simulink library "mbd_s32k1xx_ec_toolbox"  (Simulink 9.0)
settings: Solver=FixedStepDiscrete  StartTime=0.0  StopTime=10.0  FixedStep=0.1  RelTol=1e-3  EnableMultiTasking=on
InitFcn:
  | mbd_s32k_consistency_checks(bdroot(gcs));
(part 8 of 8)

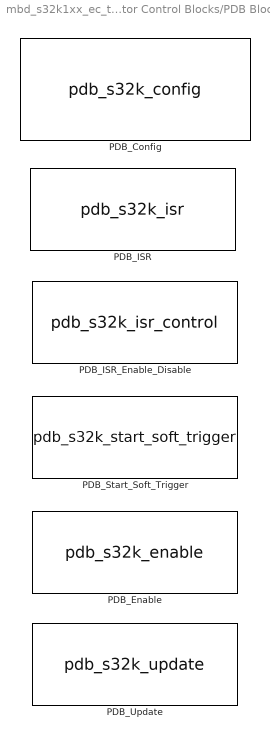
== system mbd_s32k1xx_ec_toolbox/Motor Control Blocks/PDB Blocks ==
  PDB_Config : S-Function  FunctionName=pdb_s32k_config  Parameters=funcParams  SFunctionDeploymentMode=off  EnableBusSupport=off  mask(pdb_s32k_config_block){pdbModule=0, regScCont=One-Shot, regScTrgsel=External (TRGMUX_PDB_TRIG), trgMuxSel=Trigger function is disabled, trgMuxSelPin=PTB5: [TRGMUX_IN0 | Trigger Mux Input], regModModulus=0, regScPrescaler=1, regScMult=1, regPoenPoen0=off, regPo0DlyDly1=0, regPo0DlyDly2=0, enable_pdb_init=on, show_adv_opts=on, regCh0C1En0=off, regCh0C1En1=off, regCh0C1En2=off, regCh0C1En3=off, regCh0C1En4=off, regCh0C1En5=off, regCh0C1En6=off, regCh0C1En7=off, regCh0C1Bb0=off, regCh0C1Bb1=off, regCh0C1Bb2=off, regCh0C1Bb3=off, regCh0C1Bb4=off, regCh0C1Bb5=off, regCh0C1Bb6=off, regCh0C1Bb7=off, regCh0C1Tos0=Pre-trigger is in delay mode, regCh0C1Tos1=Pre-trigger is in delay mode, regCh0C1Tos2=Pre-trigger is in delay mode, regCh0C1Tos3=Pre-trigger is in delay mode, regCh0C1Tos4=Pre-trigger is in delay mode, regCh0C1Tos5=Pre-trigger is in delay mode, regCh0C1Tos6=Pre-trigger is in delay mode, regCh0C1Tos7=Pre-trigger is in delay mode, regCh0DlyDly0=0, regCh0DlyDly1=200, regCh0DlyDly2=0, regCh0DlyDly3=0, regCh0DlyDly4=0, regCh0DlyDly5=0, regCh0DlyDly6=0, regCh0DlyDly7=0, regCh1C1En0=off, regCh1C1En1=off, regCh1C1En2=off, regCh1C1En3=off, regCh1C1En4=off, regCh1C1En5=off, regCh1C1En6=off, regCh1C1En7=off, regCh1C1Bb0=off, regCh1C1Bb1=off, regCh1C1Bb2=off, regCh1C1Bb3=off, regCh1C1Bb4=off, regCh1C1Bb5=off, regCh1C1Bb6=off, regCh1C1Bb7=off, regCh1C1Tos0=Pre-trigger is in delay mode, regCh1C1Tos1=Pre-trigger is in delay mode, regCh1C1Tos2=Pre-trigger is in delay mode, regCh1C1Tos3=Pre-trigger is in delay mode, regCh1C1Tos4=Pre-trigger is in delay mode, regCh1C1Tos5=Pre-trigger is in delay mode, regCh1C1Tos6=Pre-trigger is in delay mode, regCh1C1Tos7=Pre-trigger is in delay mode, regCh1DlyDly0=0, regCh1DlyDly1=0, regCh1DlyDly2=0, regCh1DlyDly3=0, regCh1DlyDly4=0, regCh1DlyDly5=0, regCh1DlyDly6=0, regCh1DlyDly7=0}
      mask prompts: pdbModule "Module"; regScCont "Operation Mode"; regScTrgsel "Trigger Input Source"; trgMuxSel "Input signal for External trigger"; trgMuxSelPin "Input pin for Trigger Mux Input"; regModModulus "Modulus, cycles (0 - 65535)"; regScPrescaler "Value"; regScMult "Multiplication Factor"; regPoenPoen0 "Pulse-Out0 Enable"; regPo0DlyDly1 "Pulse-Out0 Delay 1 (0 - 65535)"; regPo0DlyDly2 "Pulse-Out0 Delay 2 (0 - 65535)"; enable_pdb_init "Enable PDB in Init function"; show_adv_opts "Show Advanced Options"; regCh0C1En0 "Pre-trigger 0 Enabled"; regCh0C1En1 "Pre-trigger 1 Enabled"; regCh0C1En2 "Pre-trigger 2 Enabled"; regCh0C1En3 "Pre-trigger 3 Enabled"; regCh0C1En4 "Pre-trigger 4 Enabled"; regCh0C1En5 "Pre-trigger 5 Enabled"; regCh0C1En6 "Pre-trigger 6 Enabled"; regCh0C1En7 "Pre-trigger 7 Enabled"; regCh0C1Bb0 "Pre-trigger 0 Back-to-Back Enabled"; regCh0C1Bb1 "Pre-trigger 1 Back-to-Back Enabled"; regCh0C1Bb2 "Pre-trigger 2 Back-to-Back Enabled"; regCh0C1Bb3 "Pre-trigger 3 Back-to-Back Enabled"; regCh0C1Bb4 "Pre-trigger 4 Back-to-Back Enabled"; regCh0C1Bb5 "Pre-trigger 5 Back-to-Back Enabled"; regCh0C1Bb6 "Pre-trigger 6 Back-to-Back Enabled"; regCh0C1Bb7 "Pre-trigger 7 Back-to-Back Enabled"; regCh0C1Tos0 "Pre-Trigger 0 Output Select"; regCh0C1Tos1 "Pre-Trigger 1 Output Select"; regCh0C1Tos2 "Pre-Trigger 2 Output Select"; regCh0C1Tos3 "Pre-Trigger 3 Output Select"; regCh0C1Tos4 "Pre-Trigger 4 Output Select"; regCh0C1Tos5 "Pre-Trigger 5 Output Select"; regCh0C1Tos6 "Pre-Trigger 6 Output Select"; regCh0C1Tos7 "Pre-Trigger 7 Output Select"; regCh0DlyDly0 "Delay 0, cycles (0 - 65535)"; regCh0DlyDly1 "Delay 1, cycles (0 - 65535)"; regCh0DlyDly2 "Delay 2, cycles (0 - 65535)"; regCh0DlyDly3 "Delay 3, cycles (0 - 65535)"; regCh0DlyDly4 "Delay 4, cycles (0 - 65535)"; regCh0DlyDly5 "Delay 5, cycles (0 - 65535)"; regCh0DlyDly6 "Delay 6, cycles (0 - 65535)"; regCh0DlyDly7 "Delay 7, cycles (0 - 65535)"; regCh1C1En0 "Pre-trigger 0 Enabled"; regCh1C1En1 "Pre-trigger 1 Enabled"; regCh1C1En2 "Pre-trigger 2 Enabled"; regCh1C1En3 "Pre-trigger 3 Enabled"; regCh1C1En4 "Pre-trigger 4 Enabled"; regCh1C1En5 "Pre-trigger 5 Enabled"; regCh1C1En6 "Pre-trigger 6 Enabled"; regCh1C1En7 "Pre-trigger 7 Enabled"; regCh1C1Bb0 "Pre-trigger 0 Back-to-Back Enabled"; regCh1C1Bb1 "Pre-trigger 1 Back-to-Back Enabled"; regCh1C1Bb2 "Pre-trigger 2 Back-to-Back Enabled"; regCh1C1Bb3 "Pre-trigger 3 Back-to-Back Enabled"; regCh1C1Bb4 "Pre-trigger 4 Back-to-Back Enabled"; regCh1C1Bb5 "Pre-trigger 5 Back-to-Back Enabled"; regCh1C1Bb6 "Pre-trigger 6 Back-to-Back Enabled"; regCh1C1Bb7 "Pre-trigger 7 Back-to-Back Enabled"; regCh1C1Tos0 "Pre-Trigger 0 Output Select"; regCh1C1Tos1 "Pre-Trigger 1 Output Select"; regCh1C1Tos2 "Pre-Trigger 2 Output Select"; regCh1C1Tos3 "Pre-Trigger 3 Output Select"; regCh1C1Tos4 "Pre-Trigger 4 Output Select"; regCh1C1Tos5 "Pre-Trigger 5 Output Select"; regCh1C1Tos6 "Pre-Trigger 6 Output Select"; regCh1C1Tos7 "Pre-Trigger 7 Output Select"; regCh1DlyDly0 "Delay 0, cycles (0 - 65535)"; regCh1DlyDly1 "Delay 1, cycles (0 - 65535)"; regCh1DlyDly2 "Delay 2, cycles (0 - 65535)"; regCh1DlyDly3 "Delay 3, cycles (0 - 65535)"; regCh1DlyDly4 "Delay 4, cycles (0 - 65535)"; regCh1DlyDly5 "Delay 5, cycles (0 - 65535)"; regCh1DlyDly6 "Delay 6, cycles (0 - 65535)"; regCh1DlyDly7 "Delay 7, cycles (0 - 65535)"
      mask help: This block allows user to configure the Programmable Delay Block (PDB).
      mask init:
      | mbd_s32k_pdb_display_instances();
      | 
      | [labels, maskStr] = mbd_s32k_pdb_config_init(gcb);
      | set_param(gcb, 'MaskDisplay', labels);
      | funcParams = [];
      settings: NameChangeFcn=mbd_s32k_name_check (gcb);
      mask Help: web(fullfile(mbd_s32k_block_help, 'pdb', 'pdb_config_block.html'));
      mask TypeOptions pdbModule: 0 | 1
      mask Callback pdbModule: mbd_s32k_pdb_display_instances();
      mask TypeOptions regScCont: One-Shot | Continuous
      mask TypeOptions regScTrgsel: External (TRGMUX_PDB_TRIG) | Software
      mask Callback regScTrgsel: mbd_s32k_pdb_extrg(gcb);
      mask TypeOptions trgMuxSel: Trigger function is disabled | Trigger MUX input 0 | Trigger MUX input 1 | Trigger MUX input 2 | Trigger MUX input 3 | Trigger MUX input 4 | Trigger MUX input 5 | Trigger MUX input 6 | Trigger MUX input 7 | Trigger MUX input 8 | Trigger MUX input 9 | Trigger MUX input 10 | Trigger MUX input 11 | CMP0 Output | LPIT Channel 0 | LPIT Channel 1 | LPIT Channel 2 | LPIT Channel 3 | LPTMR0 Trigger | FTM0 Initialize Trigger | FTM0 External Trigger | FTM1 Initialize Trigger | FTM1 External Trigger | FTM2 Initialize Trigger | FTM2 External Trigger | FTM3 Initialize Trigger | FTM3 External Trigger | ADC0_COCOA | ADC0_COCOB | ADC1_COCOA | ADC1_COCOB | PDB0 Channel 0 Trigger | PDB0 Pulse out | PDB1 Channel 0 Trigger | PDB1 Pulse out | RTC Alarm | RTC Seconds Counter | Flex IO Trigger 0 | Flex IO Trigger 1 | Flex IO Trigger 2 | Flex IO Trigger 3 | LPUART0 RX Data | LPUART0 TX Data | LPUART0 RX Idle | LPUART1 RX Data | LPUART1 TX Data | LPUART1 RX Idle | LPI2C0 Master Stop | LPI2C0 Slave Stop | LPI2C1 Master Stop | LPI2C1 Slave Stop | LPSPI0 Frame | LPSPI0 RX Data | LPSPI1 Frame | LPSPI1 RX Data | SIM Software Trigger
      mask Callback trgMuxSel: mbd_s32k_pdb_extrg(gcb);
      mask TypeOptions trgMuxSelPin: PTB5: [TRGMUX_IN0 | Trigger Mux Input]
      mask Callback regModModulus: mbd_s32k_pdb_check_interval(gcb, 'regModModulus');
      mask TypeOptions regScPrescaler: 1 | 2 | 4 | 8 | 16 | 32 | 64 | 128
      mask TypeOptions regScMult: 1 | 10 | 20 | 40
      mask Callback regPoenPoen0: mbd_s32k_pdb_pulse_out_enable(gcb, '0');
      mask Callback regPo0DlyDly1: mbd_s32k_pdb_check_interval(gcb, 'regPo0DlyDly1');
      mask Callback regPo0DlyDly2: mbd_s32k_pdb_check_interval(gcb, 'regPo0DlyDly2');
      mask Callback show_adv_opts: mbd_s32k_pdb_config_cbk()
      mask Callback regCh0C1En0: mbd_s32k_pdb_channel_enable(gcb, '0', '0');
      mask Callback regCh0C1En1: mbd_s32k_pdb_channel_enable(gcb, '0', '1');
      mask Callback regCh0C1En2: mbd_s32k_pdb_channel_enable(gcb, '0', '2');
      mask Callback regCh0C1En3: mbd_s32k_pdb_channel_enable(gcb, '0', '3');
      mask Callback regCh0C1En4: mbd_s32k_pdb_channel_enable(gcb, '0', '4');
      mask Callback regCh0C1En5: mbd_s32k_pdb_channel_enable(gcb, '0', '5');
      mask Callback regCh0C1En6: mbd_s32k_pdb_channel_enable(gcb, '0', '6');
      mask Callback regCh0C1En7: mbd_s32k_pdb_channel_enable(gcb, '0', '7');
      mask TypeOptions regCh0C1Tos0: Pre-trigger is in bypassed mode | Pre-trigger is in delay mode
      mask TypeOptions regCh0C1Tos1: Pre-trigger is in bypassed mode | Pre-trigger is in delay mode
      mask TypeOptions regCh0C1Tos2: Pre-trigger is in bypassed mode | Pre-trigger is in delay mode
      mask TypeOptions regCh0C1Tos3: Pre-trigger is in bypassed mode | Pre-trigger is in delay mode
      mask TypeOptions regCh0C1Tos4: Pre-trigger is in bypassed mode | Pre-trigger is in delay mode
      mask TypeOptions regCh0C1Tos5: Pre-trigger is in bypassed mode | Pre-trigger is in delay mode
      mask TypeOptions regCh0C1Tos6: Pre-trigger is in bypassed mode | Pre-trigger is in delay mode
      mask TypeOptions regCh0C1Tos7: Pre-trigger is in bypassed mode | Pre-trigger is in delay mode
      mask Callback regCh0DlyDly0: mbd_s32k_pdb_check_interval(gcb, 'regCh0DlyDly0');
      mask Callback regCh0DlyDly1: mbd_s32k_pdb_check_interval(gcb, 'regCh0DlyDly1');
      mask Callback regCh0DlyDly2: mbd_s32k_pdb_check_interval(gcb, 'regCh0DlyDly2');
      mask Callback regCh0DlyDly3: mbd_s32k_pdb_check_interval(gcb, 'regCh0DlyDly3');
      mask Callback regCh0DlyDly4: mbd_s32k_pdb_check_interval(gcb, 'regCh0DlyDly4');
      mask Callback regCh0DlyDly5: mbd_s32k_pdb_check_interval(gcb, 'regCh0DlyDly5');
      mask Callback regCh0DlyDly6: mbd_s32k_pdb_check_interval(gcb, 'regCh0DlyDly6');
      mask Callback regCh0DlyDly7: mbd_s32k_pdb_check_interval(gcb, 'regCh0DlyDly7');
      mask Callback regCh1C1En0: mbd_s32k_pdb_channel_enable(gcb, '1', '0');
      mask Callback regCh1C1En1: mbd_s32k_pdb_channel_enable(gcb, '1', '1');
      mask Callback regCh1C1En2: mbd_s32k_pdb_channel_enable(gcb, '1', '2');
      mask Callback regCh1C1En3: mbd_s32k_pdb_channel_enable(gcb, '1', '3');
      mask Callback regCh1C1En4: mbd_s32k_pdb_channel_enable(gcb, '1', '4');
      mask Callback regCh1C1En5: mbd_s32k_pdb_channel_enable(gcb, '1', '5');
      mask Callback regCh1C1En6: mbd_s32k_pdb_channel_enable(gcb, '1', '6');
      mask Callback regCh1C1En7: mbd_s32k_pdb_channel_enable(gcb, '1', '7');
      mask TypeOptions regCh1C1Tos0: Pre-trigger is in bypassed mode | Pre-trigger is in delay mode
      mask TypeOptions regCh1C1Tos1: Pre-trigger is in bypassed mode | Pre-trigger is in delay mode
      mask TypeOptions regCh1C1Tos2: Pre-trigger is in bypassed mode | Pre-trigger is in delay mode
      mask TypeOptions regCh1C1Tos3: Pre-trigger is in bypassed mode | Pre-trigger is in delay mode
      mask TypeOptions regCh1C1Tos4: Pre-trigger is in bypassed mode | Pre-trigger is in delay mode
      mask TypeOptions regCh1C1Tos5: Pre-trigger is in bypassed mode | Pre-trigger is in delay mode
      mask TypeOptions regCh1C1Tos6: Pre-trigger is in bypassed mode | Pre-trigger is in delay mode
      mask TypeOptions regCh1C1Tos7: Pre-trigger is in bypassed mode | Pre-trigger is in delay mode
      mask Callback regCh1DlyDly0: mbd_s32k_pdb_check_interval(gcb, 'regCh1DlyDly0');
      mask Callback regCh1DlyDly1: mbd_s32k_pdb_check_interval(gcb, 'regCh1DlyDly1');
      mask Callback regCh1DlyDly2: mbd_s32k_pdb_check_interval(gcb, 'regCh1DlyDly2');
      mask Callback regCh1DlyDly3: mbd_s32k_pdb_check_interval(gcb, 'regCh1DlyDly3');
      mask Callback regCh1DlyDly4: mbd_s32k_pdb_check_interval(gcb, 'regCh1DlyDly4');
      mask Callback regCh1DlyDly5: mbd_s32k_pdb_check_interval(gcb, 'regCh1DlyDly5');
      mask Callback regCh1DlyDly6: mbd_s32k_pdb_check_interval(gcb, 'regCh1DlyDly6');
      mask Callback regCh1DlyDly7: mbd_s32k_pdb_check_interval(gcb, 'regCh1DlyDly7');
      mask DialogControl Container8 Prompt: General Settings
      mask DialogControl ParameterGroupVar0 Prompt: Prescaler Configuration
      mask DialogControl ParameterGroupVar01 Prompt: Pulse-Out Configuration
      mask Display:
      | image('nxp_logo.png', 'top-right');
      | disp(maskStr);
  PDB_Enable : S-Function  Priority=2  FunctionName=pdb_s32k_enable  SFunctionDeploymentMode=off  EnableBusSupport=off  mask(pdb_s32k_enable_block){pdbModule=0, pdbAction=Enable}
      mask prompts: pdbModule "Module"; pdbAction "Action"
      mask help: This block allows user to enable PDB block (sets PDBEN bit; if this block is not used, PDB counter is off).
      mask init:
      | maskStr = mbd_s32k_pdb_enable_to_string();
      | mbd_s32k_pdb_display_instances();
      settings: NameChangeFcn=mbd_s32k_name_check (gcb);
      mask Help: web(fullfile(mbd_s32k_block_help, 'pdb', 'pdb_enable_block.html'));
      mask TypeOptions pdbModule: 0 | 1
      mask Callback pdbModule: mbd_s32k_pdb_display_instances();
      mask TypeOptions pdbAction: Enable | Disable
      mask Display:
      | image('nxp_logo.png', 'top-right');
      | 
      | disp(maskStr);
  PDB_ISR : S-Function  Priority=2  FunctionName=pdb_s32k_isr  Parameters=funcParams  SFunctionDeploymentMode=off  EnableBusSupport=off  mask(pdb_s32k_isr_block){pdbModule=0, prioInterrupt=15, regScPdbie=off, regScPdbeie=off, regIdlyIdly=0}
      mask prompts: pdbModule "Module"; prioInterrupt "ISR priority"; regScPdbie "Counter Interrupt Enable (PDBIE)"; regScPdbeie "Sequence Error Interrupt Enable (PDBEIE)"; regIdlyIdly "Interrupt Delay, cycles (0 - 65535)"
      mask help: This block allows call user function on PDB Interrupt (when the counter value is equal to the IDLY register) or on PDB Sequence Error Interrupt.
      mask init:
      | mbd_s32k_pdb_display_instances();
      | mbd_s32k_isr_priority_cbk(gcb, 'prioInterrupt');
      | 
      | [labels, maskStr] = mbd_s32k_pdb_isr_init(gcb);
      | set_param(gcb, 'MaskDisplay', labels);
      | funcParams = [];
      settings: NameChangeFcn=mbd_s32k_name_check (gcb);
      mask Help: web(fullfile(mbd_s32k_block_help, 'pdb', 'pdb_isr_block.html'));
      mask TypeOptions pdbModule: 0 | 1
      mask Callback pdbModule: mbd_s32k_pdb_display_instances();
      mask TypeOptions prioInterrupt: 0 | 1 | 2 | 3 | 4 | 5 | 6 | 7 | 8 | 9 | 10 | 11 | 12 | 13 | 14 | 15
      mask Callback regIdlyIdly: mbd_s32k_pdb_check_interval(gcb, 'regIdlyIdly');
      mask Display:
      | image('nxp_logo.png', 'top-right');
      | port_label('output', 1, 'ISR');
      | port_label('output', 2, 'SC[PDBIF]');
      | port_label('output', 3, 'CH0S[ERRm]');
      | port_label('output', 4, 'CH1S[ERRm]');
      | disp(maskStr);
  PDB_ISR_Enable_Disable : S-Function  Priority=4  FunctionName=pdb_s32k_isr_control  Parameters=funcParams  SFunctionDeploymentMode=off  EnableBusSupport=off  mask(pdb_s32k_isr_control_block){pdbModule=0, regScPdbie=off, regScPdbeie=off}
      mask prompts: pdbModule "Module"; regScPdbie "Counter Interrupt Enable (PDBIE)"; regScPdbeie "Sequence Error Interrupt Enable (PDBEIE)"
      mask help: This block is allow to enable or disable PDB interrupts.
      mask init:
      | labels = ['image(''nxp_logo.png'', ''top-right'');', newline];
      | 
      | % Make params for s function
      | funcParams = [];
      | 
      | maskStr = [ 'PDB ISR Disable Enable Block', newline, newline, ...
      |     'Module:  ', num2str(pdbModule - 1), newline, ... 
      |     'Counter Interrupt: ', get_param(gcb,'regScPdbie'), newline, ... 
      |     'Sequence Error Interrupt: ', get_param(gcb,'regScPdbeie')];
      | 
      | mbd_s32k_pdb_display_instances();
      settings: NameChangeFcn=mbd_s32k_name_check (gcb);
      mask Help: web(fullfile(mbd_s32k_block_help, 'pdb', 'pdb_isr_control_block.html'));
      mask TypeOptions pdbModule: 0 | 1
      mask Callback pdbModule: mbd_s32k_pdb_display_instances();
      mask Display:
      | image('nxp_logo.png', 'top-right');
      | disp(maskStr);
  PDB_Start_Soft_Trigger : S-Function  Priority=3  FunctionName=pdb_s32k_start_soft_trigger  Parameters=funcParams  SFunctionDeploymentMode=off  EnableBusSupport=off  mask(pdb_s32k_start_soft_trigger_block){pdbModule=0}
      mask prompts: pdbModule "Module"
      mask help: When PDB is enabled and the software trigger is selected as the trigger input source, this block allows resets and restarts of the PDB counter.
      mask init:
      | mbd_s32k_pdb_display_instances();
      | % Make params for s function
      | funcParams = [int32(pdbModule - 1)];
      | 
      | maskStr = [ 'PDB Start Software Trigger Block', newline, newline, ...
      |     'Module:  ', num2str(pdbModule - 1)];
      settings: NameChangeFcn=mbd_s32k_name_check (gcb);
      mask Help: web(fullfile(mbd_s32k_block_help, 'pdb', 'pdb_start_soft_trigger_block.html'));
      mask TypeOptions pdbModule: 0 | 1
      mask Callback pdbModule: mbd_s32k_pdb_display_instances();
      mask Display:
      | image('nxp_logo.png', 'top-right');
      | disp(maskStr);
  PDB_Update : S-Function  Priority=2  FunctionName=pdb_s32k_update  Parameters=funcParams, funcParamNumberOfInputs  SFunctionDeploymentMode=off  EnableBusSupport=off  mask(pdb_s32k_update_block){pdbModule=0, regScLdmod=Immediately, inputModEn=off, inputIdlyEn=off, inputCh0DlyEn=off, inputCh1DlyEn=off, inputPo0DlyEn=off}
      mask prompts: pdbModule "Module"; regScLdmod "Load Mode Select"; inputModEn "Modulus input enable"; inputIdlyEn "Interrupt Delay input enable"; inputCh0DlyEn "Ch0 Delay inputs enable"; inputCh1DlyEn "Ch1 Delay inputs enable"; inputPo0DlyEn "Pulse-Out 0 Delay inputs enable"
      mask help: This block allows user to update the MOD, IDLY, CHnDLYm, INTx, and POyDLY registers, after 1 is written to LDOK.
      mask init:
      | mbd_s32k_pdb_display_instances();
      | 
      | [labels, maskStr, funcParamNumberOfInputs] = mbd_s32k_pdb_update_init(gcb);
      | set_param(gcb, 'MaskDisplay', labels);
      | funcParams = [];
      settings: NameChangeFcn=mbd_s32k_name_check (gcb);
      mask Help: web(fullfile(mbd_s32k_block_help, 'pdb', 'pdb_update_block.html'));
      mask TypeOptions pdbModule: 0 | 1
      mask Callback pdbModule: mbd_s32k_pdb_display_instances();
      mask TypeOptions regScLdmod: Immediately | PDB counter reaches the MOD register value | Trigger input event is detected | PDB counter reaches the MOD register value or a trigger input event is detected
      mask Display:
      | image('nxp_logo.png', 'top-right');
      | disp(maskStr);

== system mbd_s32k1xx_ec_toolbox/Communication Blocks/FlexIO Blocks /FlexIO I2C Blocks ==
  "FlexIO_I2C_Master_Config " : S-Function  FunctionName=flexio_i2c_master_s32k_config  SFunctionDeploymentMode=off  EnableBusSupport=off  mask(flexio_i2c_s32k_master_config){InstanceNumber=0, DriverType=Polling, BaudRate=0, SDA_pin=PTD0: [FXIO_D0 | FlexIO Bi-directional Shift/timer I/O], SCL_pin=PTD1: [FXIO_D1 | FlexIO Bi-directional Shift/timer I/O]}
      mask prompts: InstanceNumber "Instance"; DriverType "Mode"; BaudRate "Baud Rate"; SDA_pin "SDA pin"; SCL_pin "SCL pin"
      mask help: This block allows the user to configure the FlexIO module to emulate I2C communication (master mode).
      mask init:
      | maskStr = mbd_s32k_flexio_i2c_master_string();
      | mbd_s32k_flexio_i2c_master_pin_display();
      settings: NameChangeFcn=mbd_s32k_name_check(gcb);
      mask Help: web(fullfile(mbd_s32k_block_help, 'flexio', 'flexio_i2c_master_config.html'));
      mask TypeOptions InstanceNumber: 0 | 1
      mask Callback InstanceNumber: mbd_s32k_flexio_i2c_master_pin_display();
      mask TypeOptions DriverType: Polling | Interrupts
      mask TypeOptions SDA_pin: PTA10: [FXIO_D0 | FlexIO Bi-directional Shift/timer I/O] | PTA21: [FXIO_D0 | FlexIO Bi-directional Shift/timer I/O] | PTC30: [FXIO_D0 | FlexIO Bi-directional Shift/timer I/O] | PTD0: [FXIO_D0 | FlexIO Bi-directional Shift/timer I/O] | PTD9: [FXIO_D0 | FlexIO Bi-directional Shift/timer I/O] | PTA11: [FXIO_D1 | FlexIO Bi-directional Shift/timer I/O] | PTA22: [FXIO_D1 | FlexIO Bi-directional Shift/timer I/O] | PTC31: [FXIO_D1 | FlexIO Bi-directional Shift/timer I/O] | PTD1: [FXIO_D1 | FlexIO Bi-directional Shift/timer I/O] | PTD8: [FXIO_D1 | FlexIO Bi-directional Shift/timer I/O] | PTA0: [FXIO_D2 | FlexIO Bi-directional Shift/timer I/O] | PTA23: [FXIO_D2 | FlexIO Bi-directional Shift/timer I/O] | PTD18: [FXIO_D2 | FlexIO Bi-directional Shift/timer I/O] | PTE15: [FXIO_D2 | FlexIO Bi-directional Shift/timer I/O] | PTA1: [FXIO_D3 | FlexIO Bi-directional Shift/timer I/O] | PTA24: [FXIO_D3 | FlexIO Bi-directional Shift/timer I/O] | PTD19: [FXIO_D3 | FlexIO Bi-directional Shift/timer I/O] | PTE16: [FXIO_D3 | FlexIO Bi-directional Shift/timer I/O] | PTA2: [FXIO_D4 | FlexIO Bi-directional Shift/timer I/O] | PTD2: [FXIO_D4 | FlexIO Bi-directional Shift/timer I/O] | PTE10: [FXIO_D4 | FlexIO Bi-directional Shift/timer I/O] | PTE18: [FXIO_D4 | FlexIO Bi-directional Shift/timer I/O] | PTA3: [FXIO_D5 | FlexIO Bi-directional Shift/timer I/O] | PTD3: [FXIO_D5 | FlexIO Bi-directional Shift/timer I/O] | PTE11: [FXIO_D5 | FlexIO Bi-directional Shift/timer I/O] | PTE17: [FXIO_D5 | FlexIO Bi-directional Shift/timer I/O] | PTA8: [FXIO_D6 | FlexIO Bi-directional Shift/timer I/O] | PTD2: [FXIO_D6 | FlexIO Bi-directional Shift/timer I/O] | PTD31: [FXIO_D6 | FlexIO Bi-directional Shift/timer I/O] | PTE4: [FXIO_D6 | FlexIO Bi-directional Shift/timer I/O] | PTA9: [FXIO_D7 | FlexIO Bi-directional Shift/timer I/O] | PTD3: [FXIO_D7 | FlexIO Bi-directional Shift/timer I/O] | PTD26: [FXIO_D7 | FlexIO Bi-directional Shift/timer I/O] | PTE5: [FXIO_D7 | FlexIO Bi-directional Shift/timer I/O]
      mask TypeOptions SCL_pin: PTA10: [FXIO_D0 | FlexIO Bi-directional Shift/timer I/O] | PTA21: [FXIO_D0 | FlexIO Bi-directional Shift/timer I/O] | PTC30: [FXIO_D0 | FlexIO Bi-directional Shift/timer I/O] | PTD0: [FXIO_D0 | FlexIO Bi-directional Shift/timer I/O] | PTD9: [FXIO_D0 | FlexIO Bi-directional Shift/timer I/O] | PTA11: [FXIO_D1 | FlexIO Bi-directional Shift/timer I/O] | PTA22: [FXIO_D1 | FlexIO Bi-directional Shift/timer I/O] | PTC31: [FXIO_D1 | FlexIO Bi-directional Shift/timer I/O] | PTD1: [FXIO_D1 | FlexIO Bi-directional Shift/timer I/O] | PTD8: [FXIO_D1 | FlexIO Bi-directional Shift/timer I/O] | PTA0: [FXIO_D2 | FlexIO Bi-directional Shift/timer I/O] | PTA23: [FXIO_D2 | FlexIO Bi-directional Shift/timer I/O] | PTD18: [FXIO_D2 | FlexIO Bi-directional Shift/timer I/O] | PTE15: [FXIO_D2 | FlexIO Bi-directional Shift/timer I/O] | PTA1: [FXIO_D3 | FlexIO Bi-directional Shift/timer I/O] | PTA24: [FXIO_D3 | FlexIO Bi-directional Shift/timer I/O] | PTD19: [FXIO_D3 | FlexIO Bi-directional Shift/timer I/O] | PTE16: [FXIO_D3 | FlexIO Bi-directional Shift/timer I/O] | PTA2: [FXIO_D4 | FlexIO Bi-directional Shift/timer I/O] | PTD2: [FXIO_D4 | FlexIO Bi-directional Shift/timer I/O] | PTE10: [FXIO_D4 | FlexIO Bi-directional Shift/timer I/O] | PTE18: [FXIO_D4 | FlexIO Bi-directional Shift/timer I/O] | PTA3: [FXIO_D5 | FlexIO Bi-directional Shift/timer I/O] | PTD3: [FXIO_D5 | FlexIO Bi-directional Shift/timer I/O] | PTE11: [FXIO_D5 | FlexIO Bi-directional Shift/timer I/O] | PTE17: [FXIO_D5 | FlexIO Bi-directional Shift/timer I/O] | PTA8: [FXIO_D6 | FlexIO Bi-directional Shift/timer I/O] | PTD2: [FXIO_D6 | FlexIO Bi-directional Shift/timer I/O] | PTD31: [FXIO_D6 | FlexIO Bi-directional Shift/timer I/O] | PTE4: [FXIO_D6 | FlexIO Bi-directional Shift/timer I/O] | PTA9: [FXIO_D7 | FlexIO Bi-directional Shift/timer I/O] | PTD3: [FXIO_D7 | FlexIO Bi-directional Shift/timer I/O] | PTD26: [FXIO_D7 | FlexIO Bi-directional Shift/timer I/O] | PTE5: [FXIO_D7 | FlexIO Bi-directional Shift/timer I/O]
      mask DialogControl TextBaudRate Prompt: Maximum Baud Rate is FlexIO Clock / 6 = (1 300 000 Hz)
      mask Display:
      | disp(maskStr);
      | image('nxp_logo.png', 'top-right');
  FlexIO_I2C_Master_Receive : S-Function  FunctionName=flexio_i2c_master_s32k_receive  SFunctionDeploymentMode=off  EnableBusSupport=off  mask(flexio_i2c_s32k_master_receive){InstanceNumber=0, Timeout=10}
      mask prompts: InstanceNumber "Instance"; Timeout "Timeout (ms)"
      mask help: This block allows the master to receive data from slave
      mask init:
      | maskStr = 'FlexIO I2C Master Receive';
      | sFuncParams = [
      |     InstanceNumber,
      |     Timeout];
      settings: NameChangeFcn=mbd_s32k_name_check(gcb);
      mask Help: web(fullfile(mbd_s32k_block_help, 'flexio', 'flexio_i2c_master_receive.html'));
      mask TypeOptions InstanceNumber: 0 | 1
      mask Display:
      | port_label('output', 1, 'Data');
      | port_label('input',1,'Address');
      | port_label('input',2,'Length');
      | disp(maskStr);
      | image('nxp_logo.png', 'top-right');
  FlexIO_I2C_Master_Receive_ISR : S-Function  FunctionName=flexio_i2c_master_s32k_receive_isr  SFunctionDeploymentMode=off  EnableBusSupport=off  mask(flexio_i2c_s32k_master_receive_isr){InstanceNumber=0}
      mask prompts: InstanceNumber "Instance"
      mask help: This block allows the master to receive data from slave
      mask init:
      | maskStr = 'FlexIO I2C Master Receive ISR';
      | 
      | sFuncParams = [
      |     InstanceNumber];
      settings: NameChangeFcn=mbd_s32k_name_check(gcb);
      mask Help: web(fullfile(mbd_s32k_block_help, 'flexio', 'flexio_i2c_master_receive_isr.html'));
      mask TypeOptions InstanceNumber: 0 | 1
      mask Display:
      | disp(maskStr)
      | port_label('output', 1, 'Trigger');
      | port_label('output', 2, 'Data');
      | port_label('input',1,'Address');
      | port_label('input',2,'Length');
      | image('nxp_logo.png', 'top-right');
  FlexIO_I2C_Master_Transmit : S-Function  FunctionName=flexio_i2c_master_s32k_transmit  SFunctionDeploymentMode=off  EnableBusSupport=off  mask(flexio_i2c_s32k_master_transmit){InstanceNumber=0, Timeout=10}
      mask prompts: InstanceNumber "Instance"; Timeout "Timeout (ms)"
      mask help: This block allows the master to transmit data to slave
      mask init:
      | maskStr = 'FlexIO I2C Master Transmit';
      | 
      | sFuncParams = [
      |     InstanceNumber
      |     Timeout];
      settings: NameChangeFcn=mbd_s32k_name_check(gcb);
      mask Help: web(fullfile(mbd_s32k_block_help, 'flexio', 'flexio_i2c_master_transmit.html'));
      mask TypeOptions InstanceNumber: 0 | 1
      mask Display:
      | port_label('input', 1, 'Data');
      | port_label('input', 2, 'SendStop');
      | port_label('input', 3, 'Address');
      | disp(maskStr);
      | image('nxp_logo.png', 'top-right');
  FlexIO_I2C_Master_Transmit_ISR : S-Function  FunctionName=flexio_i2c_master_s32k_transmit_isr  SFunctionDeploymentMode=off  EnableBusSupport=off  mask(flexio_i2c_s32k_master_transmit_isr){InstanceNumber=0}
      mask prompts: InstanceNumber "Instance"
      mask help: This block allows the master to transmit data to slave
      mask init:
      | maskStr = 'FlexIO I2C Master Transmit ISR';
      | 
      | sFuncParams = [
      |     InstanceNumber];
      settings: NameChangeFcn=mbd_s32k_name_check(gcb);
      mask Help: web(fullfile(mbd_s32k_block_help, 'flexio', 'flexio_i2c_master_transmit_isr.html'));
      mask TypeOptions InstanceNumber: 0 | 1
      mask Display:
      | disp(maskStr)
      | port_label('input', 1, 'Data');
      | port_label('input', 2, 'SendStop');
      | port_label('input', 3, 'Address');
      | port_label('output',1,'Trigger');
      | image('nxp_logo.png', 'top-right');

== system mbd_s32k1xx_ec_toolbox/Communication Blocks/FlexIO Blocks /FlexIO SPI Blocks ==
  "FlexIO_SPI_Config " : S-Function  FunctionName=flexio_spi_s32k_config  SFunctionDeploymentMode=off  EnableBusSupport=off  mask(flexio_spi_s32k_config){InstanceNumber=0, Role=Slave, DriverType=Polling, BaudRate=100000, ShowAdvanced=on, MOSIPin=PTD0: [FXIO_D0 | FlexIO Bi-directional Shift/timer I/O], MISOPin=PTD1: [FXIO_D1 | FlexIO Bi-directional Shift/timer I/O], SCKPin=PTE15: [FXIO_D2 | FlexIO Bi-directional Shift/timer I/O], SSPin=PTE16: [FXIO_D3 | FlexIO Bi-directional Shift/timer I/O], CPHA=0, CPOL=0, BitOrder=MSB first, TransferSize=1B}
      mask prompts: InstanceNumber "Instance"; DriverType "Mode"; BaudRate "Baud Rate"; ShowAdvanced "Show advanced options"; MOSIPin "MOSI pin"; MISOPin "MISO pin"; SCKPin "SCK pin"; SSPin "SS pin"; BitOrder "Bit order"; TransferSize "Transfer size"
      mask help: This block allows the user to configure the FlexIO module to emulate spi communication.
      mask init:
      | maskStr = mbd_s32k_flexio_spi_string();
      | mbd_s32k_flexio_spi_pin_display();
      settings: NameChangeFcn=mbd_s32k_name_check(gcb);
      mask Help: web(fullfile(mbd_s32k_block_help, 'flexio', 'flexio_spi_config.html'));
      mask TypeOptions InstanceNumber: 0 | 1
      mask Callback InstanceNumber: mbd_s32k_flexio_spi_pin_display()
      mask TypeOptions Role: Master | Slave
      mask Callback Role: mbd_s32k_flexio_spi_config_cbk
      mask TypeOptions DriverType: Polling | Interrupts
      mask Callback ShowAdvanced: mbd_s32k_flexio_spi_config_cbk()
      mask TypeOptions MOSIPin: PTA10: [FXIO_D0 | FlexIO Bi-directional Shift/timer I/O] | PTA21: [FXIO_D0 | FlexIO Bi-directional Shift/timer I/O] | PTC30: [FXIO_D0 | FlexIO Bi-directional Shift/timer I/O] | PTD0: [FXIO_D0 | FlexIO Bi-directional Shift/timer I/O] | PTD9: [FXIO_D0 | FlexIO Bi-directional Shift/timer I/O] | PTA11: [FXIO_D1 | FlexIO Bi-directional Shift/timer I/O] | PTA22: [FXIO_D1 | FlexIO Bi-directional Shift/timer I/O] | PTC31: [FXIO_D1 | FlexIO Bi-directional Shift/timer I/O] | PTD1: [FXIO_D1 | FlexIO Bi-directional Shift/timer I/O] | PTD8: [FXIO_D1 | FlexIO Bi-directional Shift/timer I/O] | PTA0: [FXIO_D2 | FlexIO Bi-directional Shift/timer I/O] | PTA23: [FXIO_D2 | FlexIO Bi-directional Shift/timer I/O] | PTD18: [FXIO_D2 | FlexIO Bi-directional Shift/timer I/O] | PTE15: [FXIO_D2 | FlexIO Bi-directional Shift/timer I/O] | PTA1: [FXIO_D3 | FlexIO Bi-directional Shift/timer I/O] | PTA24: [FXIO_D3 | FlexIO Bi-directional Shift/timer I/O] | PTD19: [FXIO_D3 | FlexIO Bi-directional Shift/timer I/O] | PTE16: [FXIO_D3 | FlexIO Bi-directional Shift/timer I/O] | PTA2: [FXIO_D4 | FlexIO Bi-directional Shift/timer I/O] | PTD2: [FXIO_D4 | FlexIO Bi-directional Shift/timer I/O] | PTE10: [FXIO_D4 | FlexIO Bi-directional Shift/timer I/O] | PTE18: [FXIO_D4 | FlexIO Bi-directional Shift/timer I/O] | PTA3: [FXIO_D5 | FlexIO Bi-directional Shift/timer I/O] | PTD3: [FXIO_D5 | FlexIO Bi-directional Shift/timer I/O] | PTE11: [FXIO_D5 | FlexIO Bi-directional Shift/timer I/O] | PTE17: [FXIO_D5 | FlexIO Bi-directional Shift/timer I/O] | PTA8: [FXIO_D6 | FlexIO Bi-directional Shift/timer I/O] | PTD2: [FXIO_D6 | FlexIO Bi-directional Shift/timer I/O] | PTD31: [FXIO_D6 | FlexIO Bi-directional Shift/timer I/O] | PTE4: [FXIO_D6 | FlexIO Bi-directional Shift/timer I/O] | PTA9: [FXIO_D7 | FlexIO Bi-directional Shift/timer I/O] | PTD3: [FXIO_D7 | FlexIO Bi-directional Shift/timer I/O] | PTD26: [FXIO_D7 | FlexIO Bi-directional Shift/timer I/O] | PTE5: [FXIO_D7 | FlexIO Bi-directional Shift/timer I/O]
      mask TypeOptions MISOPin: PTA10: [FXIO_D0 | FlexIO Bi-directional Shift/timer I/O] | PTA21: [FXIO_D0 | FlexIO Bi-directional Shift/timer I/O] | PTC30: [FXIO_D0 | FlexIO Bi-directional Shift/timer I/O] | PTD0: [FXIO_D0 | FlexIO Bi-directional Shift/timer I/O] | PTD9: [FXIO_D0 | FlexIO Bi-directional Shift/timer I/O] | PTA11: [FXIO_D1 | FlexIO Bi-directional Shift/timer I/O] | PTA22: [FXIO_D1 | FlexIO Bi-directional Shift/timer I/O] | PTC31: [FXIO_D1 | FlexIO Bi-directional Shift/timer I/O] | PTD1: [FXIO_D1 | FlexIO Bi-directional Shift/timer I/O] | PTD8: [FXIO_D1 | FlexIO Bi-directional Shift/timer I/O] | PTA0: [FXIO_D2 | FlexIO Bi-directional Shift/timer I/O] | PTA23: [FXIO_D2 | FlexIO Bi-directional Shift/timer I/O] | PTD18: [FXIO_D2 | FlexIO Bi-directional Shift/timer I/O] | PTE15: [FXIO_D2 | FlexIO Bi-directional Shift/timer I/O] | PTA1: [FXIO_D3 | FlexIO Bi-directional Shift/timer I/O] | PTA24: [FXIO_D3 | FlexIO Bi-directional Shift/timer I/O] | PTD19: [FXIO_D3 | FlexIO Bi-directional Shift/timer I/O] | PTE16: [FXIO_D3 | FlexIO Bi-directional Shift/timer I/O] | PTA2: [FXIO_D4 | FlexIO Bi-directional Shift/timer I/O] | PTD2: [FXIO_D4 | FlexIO Bi-directional Shift/timer I/O] | PTE10: [FXIO_D4 | FlexIO Bi-directional Shift/timer I/O] | PTE18: [FXIO_D4 | FlexIO Bi-directional Shift/timer I/O] | PTA3: [FXIO_D5 | FlexIO Bi-directional Shift/timer I/O] | PTD3: [FXIO_D5 | FlexIO Bi-directional Shift/timer I/O] | PTE11: [FXIO_D5 | FlexIO Bi-directional Shift/timer I/O] | PTE17: [FXIO_D5 | FlexIO Bi-directional Shift/timer I/O] | PTA8: [FXIO_D6 | FlexIO Bi-directional Shift/timer I/O] | PTD2: [FXIO_D6 | FlexIO Bi-directional Shift/timer I/O] | PTD31: [FXIO_D6 | FlexIO Bi-directional Shift/timer I/O] | PTE4: [FXIO_D6 | FlexIO Bi-directional Shift/timer I/O] | PTA9: [FXIO_D7 | FlexIO Bi-directional Shift/timer I/O] | PTD3: [FXIO_D7 | FlexIO Bi-directional Shift/timer I/O] | PTD26: [FXIO_D7 | FlexIO Bi-directional Shift/timer I/O] | PTE5: [FXIO_D7 | FlexIO Bi-directional Shift/timer I/O]
      mask TypeOptions SCKPin: PTA10: [FXIO_D0 | FlexIO Bi-directional Shift/timer I/O] | PTA21: [FXIO_D0 | FlexIO Bi-directional Shift/timer I/O] | PTC30: [FXIO_D0 | FlexIO Bi-directional Shift/timer I/O] | PTD0: [FXIO_D0 | FlexIO Bi-directional Shift/timer I/O] | PTD9: [FXIO_D0 | FlexIO Bi-directional Shift/timer I/O] | PTA11: [FXIO_D1 | FlexIO Bi-directional Shift/timer I/O] | PTA22: [FXIO_D1 | FlexIO Bi-directional Shift/timer I/O] | PTC31: [FXIO_D1 | FlexIO Bi-directional Shift/timer I/O] | PTD1: [FXIO_D1 | FlexIO Bi-directional Shift/timer I/O] | PTD8: [FXIO_D1 | FlexIO Bi-directional Shift/timer I/O] | PTA0: [FXIO_D2 | FlexIO Bi-directional Shift/timer I/O] | PTA23: [FXIO_D2 | FlexIO Bi-directional Shift/timer I/O] | PTD18: [FXIO_D2 | FlexIO Bi-directional Shift/timer I/O] | PTE15: [FXIO_D2 | FlexIO Bi-directional Shift/timer I/O] | PTA1: [FXIO_D3 | FlexIO Bi-directional Shift/timer I/O] | PTA24: [FXIO_D3 | FlexIO Bi-directional Shift/timer I/O] | PTD19: [FXIO_D3 | FlexIO Bi-directional Shift/timer I/O] | PTE16: [FXIO_D3 | FlexIO Bi-directional Shift/timer I/O] | PTA2: [FXIO_D4 | FlexIO Bi-directional Shift/timer I/O] | PTD2: [FXIO_D4 | FlexIO Bi-directional Shift/timer I/O] | PTE10: [FXIO_D4 | FlexIO Bi-directional Shift/timer I/O] | PTE18: [FXIO_D4 | FlexIO Bi-directional Shift/timer I/O] | PTA3: [FXIO_D5 | FlexIO Bi-directional Shift/timer I/O] | PTD3: [FXIO_D5 | FlexIO Bi-directional Shift/timer I/O] | PTE11: [FXIO_D5 | FlexIO Bi-directional Shift/timer I/O] | PTE17: [FXIO_D5 | FlexIO Bi-directional Shift/timer I/O] | PTA8: [FXIO_D6 | FlexIO Bi-directional Shift/timer I/O] | PTD2: [FXIO_D6 | FlexIO Bi-directional Shift/timer I/O] | PTD31: [FXIO_D6 | FlexIO Bi-directional Shift/timer I/O] | PTE4: [FXIO_D6 | FlexIO Bi-directional Shift/timer I/O] | PTA9: [FXIO_D7 | FlexIO Bi-directional Shift/timer I/O] | PTD3: [FXIO_D7 | FlexIO Bi-directional Shift/timer I/O] | PTD26: [FXIO_D7 | FlexIO Bi-directional Shift/timer I/O] | PTE5: [FXIO_D7 | FlexIO Bi-directional Shift/timer I/O]
      mask TypeOptions SSPin: PTA10: [FXIO_D0 | FlexIO Bi-directional Shift/timer I/O] | PTA21: [FXIO_D0 | FlexIO Bi-directional Shift/timer I/O] | PTC30: [FXIO_D0 | FlexIO Bi-directional Shift/timer I/O] | PTD0: [FXIO_D0 | FlexIO Bi-directional Shift/timer I/O] | PTD9: [FXIO_D0 | FlexIO Bi-directional Shift/timer I/O] | PTA11: [FXIO_D1 | FlexIO Bi-directional Shift/timer I/O] | PTA22: [FXIO_D1 | FlexIO Bi-directional Shift/timer I/O] | PTC31: [FXIO_D1 | FlexIO Bi-directional Shift/timer I/O] | PTD1: [FXIO_D1 | FlexIO Bi-directional Shift/timer I/O] | PTD8: [FXIO_D1 | FlexIO Bi-directional Shift/timer I/O] | PTA0: [FXIO_D2 | FlexIO Bi-directional Shift/timer I/O] | PTA23: [FXIO_D2 | FlexIO Bi-directional Shift/timer I/O] | PTD18: [FXIO_D2 | FlexIO Bi-directional Shift/timer I/O] | PTE15: [FXIO_D2 | FlexIO Bi-directional Shift/timer I/O] | PTA1: [FXIO_D3 | FlexIO Bi-directional Shift/timer I/O] | PTA24: [FXIO_D3 | FlexIO Bi-directional Shift/timer I/O] | PTD19: [FXIO_D3 | FlexIO Bi-directional Shift/timer I/O] | PTE16: [FXIO_D3 | FlexIO Bi-directional Shift/timer I/O] | PTA2: [FXIO_D4 | FlexIO Bi-directional Shift/timer I/O] | PTD2: [FXIO_D4 | FlexIO Bi-directional Shift/timer I/O] | PTE10: [FXIO_D4 | FlexIO Bi-directional Shift/timer I/O] | PTE18: [FXIO_D4 | FlexIO Bi-directional Shift/timer I/O] | PTA3: [FXIO_D5 | FlexIO Bi-directional Shift/timer I/O] | PTD3: [FXIO_D5 | FlexIO Bi-directional Shift/timer I/O] | PTE11: [FXIO_D5 | FlexIO Bi-directional Shift/timer I/O] | PTE17: [FXIO_D5 | FlexIO Bi-directional Shift/timer I/O] | PTA8: [FXIO_D6 | FlexIO Bi-directional Shift/timer I/O] | PTD2: [FXIO_D6 | FlexIO Bi-directional Shift/timer I/O] | PTD31: [FXIO_D6 | FlexIO Bi-directional Shift/timer I/O] | PTE4: [FXIO_D6 | FlexIO Bi-directional Shift/timer I/O] | PTA9: [FXIO_D7 | FlexIO Bi-directional Shift/timer I/O] | PTD3: [FXIO_D7 | FlexIO Bi-directional Shift/timer I/O] | PTD26: [FXIO_D7 | FlexIO Bi-directional Shift/timer I/O] | PTE5: [FXIO_D7 | FlexIO Bi-directional Shift/timer I/O]
      mask TypeOptions CPHA: 0 | 1
      mask TypeOptions CPOL: 0 | 1
      mask TypeOptions BitOrder: MSB first | LSB first
      mask TypeOptions TransferSize: 1B | 2B | 4B
      mask Display:
      | disp(maskStr);
      | image('nxp_logo.png', 'top-right');
  FlexIO_SPI_Master_Transfer : S-Function  FunctionName=flexio_spi_s32k_master_transfer  SFunctionDeploymentMode=off  EnableBusSupport=off  mask(flexio_spi_s32k_master_transfer){InstanceNumber=0, Timeout=10}
      mask prompts: InstanceNumber "Instance"; Timeout "Timeout (ms)"
      mask help: This block allows the user to transfer data betwen master and slave.
      mask init:
      | maskStr = 'FlexIO SPI Master Transfer';
      settings: NameChangeFcn=mbd_s32k_name_check(gcb);
      mask Help: web(fullfile(mbd_s32k_block_help, 'flexio', 'flexio_spi_master_transfer.html'));
      mask TypeOptions InstanceNumber: 0 | 1
      mask Display:
      | port_label('input', 1, 'Data Tx');
      | port_label('output', 1, 'Data Rx');
      | disp(maskStr);
      | image('nxp_logo.png', 'top-right');
  FlexIO_SPI_Master_Transfer_ISR : S-Function  FunctionName=flexio_spi_s32k_master_transfer_isr  SFunctionDeploymentMode=off  EnableBusSupport=off  mask(flexio_spi_s32k_master_transfer_isr){InstanceNumber=0}
      mask prompts: InstanceNumber "Instance"
      mask help: This block allows the user to transfer data (non-blocking).
      mask init:
      | maskStr = 'FlexIO SPI Master Transfer ISR';
      settings: NameChangeFcn=mbd_s32k_name_check(gcb);
      mask Help: web(fullfile(mbd_s32k_block_help, 'flexio', 'flexio_spi_master_transfer_isr.html'));
      mask TypeOptions InstanceNumber: 0 | 1
      mask Display:
      | disp(maskStr)
      | port_label('input', 1, 'Data Tx');
      | port_label('output', 2, 'Data Rx');
      | port_label('output', 1, 'Trigger');
      | image('nxp_logo.png', 'top-right');
  FlexIO_SPI_Slave_Transfer : S-Function  FunctionName=flexio_spi_s32k_slave_transfer  SFunctionDeploymentMode=off  EnableBusSupport=off  mask(flexio_spi_s32k_slave_transfer){InstanceNumber=0, Timeout=10}
      mask prompts: InstanceNumber "Instance"; Timeout "Timeout (ms)"
      mask help: This block allows the user to transfer data (slave side).
      mask init:
      | maskStr = 'FlexIO SPI Slave Transfer';
      settings: NameChangeFcn=mbd_s32k_name_check(gcb);
      mask Help: web(fullfile(mbd_s32k_block_help, 'flexio', 'flexio_spi_slave_transfer.html'));
      mask TypeOptions InstanceNumber: 0 | 1
      mask Display:
      | port_label('output', 1, 'Data Rx');
      | port_label('input', 1, 'Data Tx');
      | disp(maskStr);
      | image('nxp_logo.png', 'top-right');
  FlexIO_SPI_Slave_Transfer_ISR : S-Function  FunctionName=flexio_spi_s32k_slave_transfer_isr  SFunctionDeploymentMode=off  EnableBusSupport=off  mask(flexio_spi_s32k_slave_transfer_isr){InstanceNumber=0}
      mask prompts: InstanceNumber "Instance"
      mask help: This block allows the user to transfer data (non-blocking).
      mask init:
      | maskStr = 'FlexIO SPI Slave Transfer ISR';
      settings: NameChangeFcn=mbd_s32k_name_check(gcb);
      mask Help: web(fullfile(mbd_s32k_block_help, 'flexio', 'flexio_spi_slave_transfer_isr.html'));
      mask TypeOptions InstanceNumber: 0 | 1
      mask Display:
      | disp(maskStr)
      | port_label('output', 1, 'Trigger');
      | port_label('output', 2, 'Data Rx');
      | port_label('input', 1, 'Data Tx');
      | image('nxp_logo.png', 'top-right');

== system mbd_s32k1xx_ec_toolbox/Communication Blocks/FlexIO Blocks /FlexIO UART Blocks ==
  "FlexIO_UART_Config " : S-Function  FunctionName=flexio_uart_s32k_config  SFunctionDeploymentMode=off  EnableBusSupport=off  mask(flexio_uart_s32k_config){InstanceNumber=0, DriverType=Polling, BitCount=8, BaudRate=115200, TxPin=PTD0: [FXIO_D0 | FlexIO Bi-directional Shift/timer I/O], RxPin=PTD1: [FXIO_D1 | FlexIO Bi-directional Shift/timer I/O]}
      mask prompts: InstanceNumber "Instance"; DriverType "Mode"; BitCount "Bit count"; BaudRate "Baud Rate"; TxPin "Tx Pin"; RxPin "Rx Pin"
      mask help: This block allows the user to configure the FlexIO module to emulate UART communication.
      mask init:
      | maskStr = mbd_s32k_flexio_uart_config_string();
      | mbd_s32k_flexio_uart_pin_display();
      settings: NameChangeFcn=mbd_s32k_name_check(gcb);
      mask Help: web(fullfile(mbd_s32k_block_help, 'flexio', 'flexio_uart_config.html'));
      mask TypeOptions InstanceNumber: 0 | 1 | 2 | 3
      mask Callback InstanceNumber: mbd_s32k_flexio_uart_pin_display();
      mask TypeOptions DriverType: Polling | Interrupts
      mask TypeOptions TxPin: PTA10: [FXIO_D0 | FlexIO Bi-directional Shift/timer I/O] | PTA21: [FXIO_D0 | FlexIO Bi-directional Shift/timer I/O] | PTC30: [FXIO_D0 | FlexIO Bi-directional Shift/timer I/O] | PTD0: [FXIO_D0 | FlexIO Bi-directional Shift/timer I/O] | PTD9: [FXIO_D0 | FlexIO Bi-directional Shift/timer I/O] | PTA11: [FXIO_D1 | FlexIO Bi-directional Shift/timer I/O] | PTA22: [FXIO_D1 | FlexIO Bi-directional Shift/timer I/O] | PTC31: [FXIO_D1 | FlexIO Bi-directional Shift/timer I/O] | PTD1: [FXIO_D1 | FlexIO Bi-directional Shift/timer I/O] | PTD8: [FXIO_D1 | FlexIO Bi-directional Shift/timer I/O] | PTA0: [FXIO_D2 | FlexIO Bi-directional Shift/timer I/O] | PTA23: [FXIO_D2 | FlexIO Bi-directional Shift/timer I/O] | PTD18: [FXIO_D2 | FlexIO Bi-directional Shift/timer I/O] | PTE15: [FXIO_D2 | FlexIO Bi-directional Shift/timer I/O] | PTA1: [FXIO_D3 | FlexIO Bi-directional Shift/timer I/O] | PTA24: [FXIO_D3 | FlexIO Bi-directional Shift/timer I/O] | PTD19: [FXIO_D3 | FlexIO Bi-directional Shift/timer I/O] | PTE16: [FXIO_D3 | FlexIO Bi-directional Shift/timer I/O] | PTA2: [FXIO_D4 | FlexIO Bi-directional Shift/timer I/O] | PTD2: [FXIO_D4 | FlexIO Bi-directional Shift/timer I/O] | PTE10: [FXIO_D4 | FlexIO Bi-directional Shift/timer I/O] | PTE18: [FXIO_D4 | FlexIO Bi-directional Shift/timer I/O] | PTA3: [FXIO_D5 | FlexIO Bi-directional Shift/timer I/O] | PTD3: [FXIO_D5 | FlexIO Bi-directional Shift/timer I/O] | PTE11: [FXIO_D5 | FlexIO Bi-directional Shift/timer I/O] | PTE17: [FXIO_D5 | FlexIO Bi-directional Shift/timer I/O] | PTA8: [FXIO_D6 | FlexIO Bi-directional Shift/timer I/O] | PTD2: [FXIO_D6 | FlexIO Bi-directional Shift/timer I/O] | PTD31: [FXIO_D6 | FlexIO Bi-directional Shift/timer I/O] | PTE4: [FXIO_D6 | FlexIO Bi-directional Shift/timer I/O] | PTA9: [FXIO_D7 | FlexIO Bi-directional Shift/timer I/O] | PTD3: [FXIO_D7 | FlexIO Bi-directional Shift/timer I/O] | PTD26: [FXIO_D7 | FlexIO Bi-directional Shift/timer I/O] | PTE5: [FXIO_D7 | FlexIO Bi-directional Shift/timer I/O]
      mask TypeOptions RxPin: PTA10: [FXIO_D0 | FlexIO Bi-directional Shift/timer I/O] | PTA21: [FXIO_D0 | FlexIO Bi-directional Shift/timer I/O] | PTC30: [FXIO_D0 | FlexIO Bi-directional Shift/timer I/O] | PTD0: [FXIO_D0 | FlexIO Bi-directional Shift/timer I/O] | PTD9: [FXIO_D0 | FlexIO Bi-directional Shift/timer I/O] | PTA11: [FXIO_D1 | FlexIO Bi-directional Shift/timer I/O] | PTA22: [FXIO_D1 | FlexIO Bi-directional Shift/timer I/O] | PTC31: [FXIO_D1 | FlexIO Bi-directional Shift/timer I/O] | PTD1: [FXIO_D1 | FlexIO Bi-directional Shift/timer I/O] | PTD8: [FXIO_D1 | FlexIO Bi-directional Shift/timer I/O] | PTA0: [FXIO_D2 | FlexIO Bi-directional Shift/timer I/O] | PTA23: [FXIO_D2 | FlexIO Bi-directional Shift/timer I/O] | PTD18: [FXIO_D2 | FlexIO Bi-directional Shift/timer I/O] | PTE15: [FXIO_D2 | FlexIO Bi-directional Shift/timer I/O] | PTA1: [FXIO_D3 | FlexIO Bi-directional Shift/timer I/O] | PTA24: [FXIO_D3 | FlexIO Bi-directional Shift/timer I/O] | PTD19: [FXIO_D3 | FlexIO Bi-directional Shift/timer I/O] | PTE16: [FXIO_D3 | FlexIO Bi-directional Shift/timer I/O] | PTA2: [FXIO_D4 | FlexIO Bi-directional Shift/timer I/O] | PTD2: [FXIO_D4 | FlexIO Bi-directional Shift/timer I/O] | PTE10: [FXIO_D4 | FlexIO Bi-directional Shift/timer I/O] | PTE18: [FXIO_D4 | FlexIO Bi-directional Shift/timer I/O] | PTA3: [FXIO_D5 | FlexIO Bi-directional Shift/timer I/O] | PTD3: [FXIO_D5 | FlexIO Bi-directional Shift/timer I/O] | PTE11: [FXIO_D5 | FlexIO Bi-directional Shift/timer I/O] | PTE17: [FXIO_D5 | FlexIO Bi-directional Shift/timer I/O] | PTA8: [FXIO_D6 | FlexIO Bi-directional Shift/timer I/O] | PTD2: [FXIO_D6 | FlexIO Bi-directional Shift/timer I/O] | PTD31: [FXIO_D6 | FlexIO Bi-directional Shift/timer I/O] | PTE4: [FXIO_D6 | FlexIO Bi-directional Shift/timer I/O] | PTA9: [FXIO_D7 | FlexIO Bi-directional Shift/timer I/O] | PTD3: [FXIO_D7 | FlexIO Bi-directional Shift/timer I/O] | PTD26: [FXIO_D7 | FlexIO Bi-directional Shift/timer I/O] | PTE5: [FXIO_D7 | FlexIO Bi-directional Shift/timer I/O]
      mask Display:
      | disp(maskStr);
      | image('nxp_logo.png', 'top-right');
  FlexIO_UART_Receive : S-Function  FunctionName=flexio_uart_s32k_receive  SFunctionDeploymentMode=off  EnableBusSupport=off  mask(flexio_uart_s32k_receive){InstanceNumber=0, Timeout=10}
      mask prompts: InstanceNumber "Instance"; Timeout "Timeout (ms)"
      mask help: This block allows the user to receive data.
      mask init:
      | maskStr = 'FlexIO UART Receive';
      | sFuncParams = [
      |     InstanceNumber,
      |     Timeout];
      settings: NameChangeFcn=mbd_s32k_name_check(gcb);
      mask Help: web(fullfile(mbd_s32k_block_help, 'flexio', 'flexio_uart_receive.html'));
      mask TypeOptions InstanceNumber: 0 | 1 | 2 | 3
      mask Display:
      | port_label('output', 1, 'Data');
      | port_label('input', 1, 'Length');
      | disp(maskStr);
      | image('nxp_logo.png', 'top-right');
  FlexIO_UART_Receive_ISR : S-Function  FunctionName=flexio_uart_s32k_receive_isr  SFunctionDeploymentMode=off  EnableBusSupport=off  mask(flexio_uart_s32k_receive_isr){InstanceNumber=0}
      mask prompts: InstanceNumber "Instance"
      mask help: This block allows the user to receive data.
      mask init:
      | maskStr = 'FlexIO UART Receive ISR';
      | 
      | sFuncParams = [
      |     InstanceNumber];
      settings: NameChangeFcn=mbd_s32k_name_check(gcb);
      mask Help: web(fullfile(mbd_s32k_block_help, 'flexio', 'flexio_uart_receive_isr.html'));
      mask TypeOptions InstanceNumber: 0 | 1 | 2 | 3
      mask Display:
      | disp(maskStr)
      | port_label('output', 1, 'Trigger');
      | port_label('output', 2, 'Data');
      | port_label('input', 1, 'Length');
      | image('nxp_logo.png', 'top-right');
  FlexIO_UART_Transmit : S-Function  FunctionName=flexio_uart_s32k_transmit  SFunctionDeploymentMode=off  EnableBusSupport=off  mask(flexio_uart_s32k_transmit){InstanceNumber=0, Timeout=10}
      mask prompts: InstanceNumber "Instance"; Timeout "Timeout (ms)"
      mask help: This block allows the user to transmit data.
      mask init:
      | maskStr = 'FlexIO UART Transmit';
      | 
      | sFuncParams = [
      |     InstanceNumber
      |     Timeout];
      settings: NameChangeFcn=mbd_s32k_name_check(gcb);
      mask Help: web(fullfile(mbd_s32k_block_help, 'flexio', 'flexio_uart_transmit.html'));
      mask TypeOptions InstanceNumber: 0 | 1 | 2 | 3
      mask Display:
      | port_label('input', 1, 'Data');
      | disp(maskStr);
      | image('nxp_logo.png', 'top-right');
  FlexIO_UART_Transmit_ISR : S-Function  FunctionName=flexio_uart_s32k_transmit_isr  SFunctionDeploymentMode=off  EnableBusSupport=off  mask(flexio_uart_s32k_transmit_isr){InstanceNumber=0}
      mask prompts: InstanceNumber "Instance"
      mask help: This block allows the user to transmit data.
      mask init:
      | maskStr = 'FlexIO UART Transmit ISR';
      | 
      | sFuncParams = [
      |     InstanceNumber];
      settings: NameChangeFcn=mbd_s32k_name_check(gcb);
      mask Help: web(fullfile(mbd_s32k_block_help, 'flexio', 'flexio_uart_transmit_isr.html'));
      mask TypeOptions InstanceNumber: 0 | 1 | 2 | 3
      mask Display:
      | disp(maskStr)
      | port_label('input', 1, 'Data');
      | port_label('output',1,'Trigger');
      | image('nxp_logo.png', 'top-right');
